simulink model "AntriebeW_V2_Heatflow_D"  (Simulink 7.6)
settings: Solver=ode45  StartTime=0.0  StopTime=SimulTime  RelTol=1e-3
values from neighbouring files (symbols this model uses):
  hsp = 200    [ParamtersAntriebeW_D.m]
  r = 0.2    [ParamtersAntriebeW_D.m]
  R = 25    [ParamtersAntriebeW_D.m]    (also in PlottingAntriebeHeatFlow.m = Scp_DrivesT.signals(3).values(:,1))
  sb = 5.67*(10^-8)    (= 5.67e-08)    [ParamtersAntriebeW_D.m]
  T_amb = 296    [ParamtersAntriebeW_D.m]
undefined symbols (not defined in the file or in its folder): A, Drive, Job, magnitude
libraries: simulink x1
settings Model: Creator=Coni  LastModifiedBy=conid

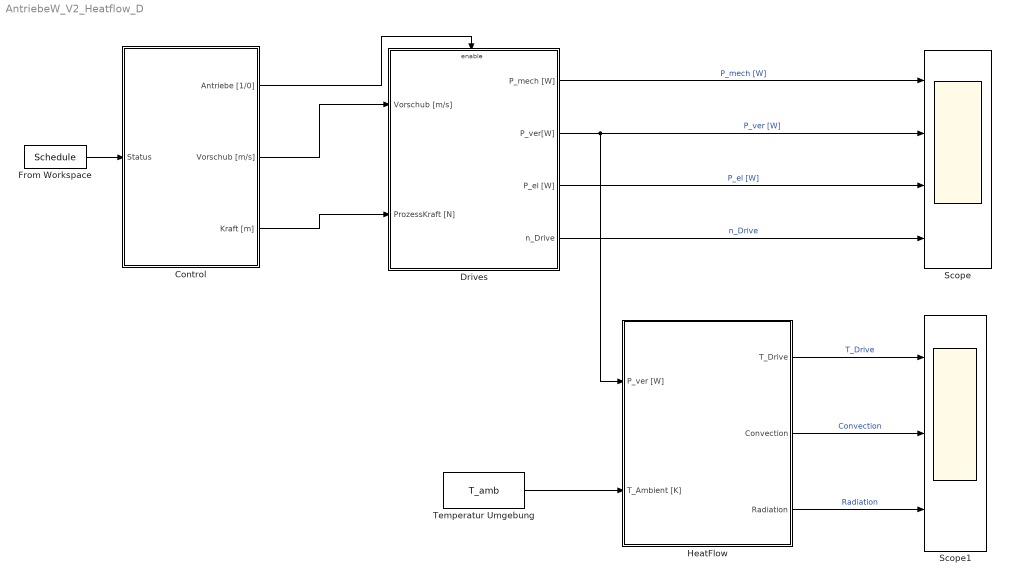
== system AntriebeW_V2_Heatflow_D ==
  Control : Subsystem  TreatAsAtomicUnit=on  mask{Antriebe=[0 1 1 1 1], Job=Job}
      mask prompts: Job "Job Struct"
      mask help:
      | Controls the components of the machine:
      |
      | Status:
      |     0. Off
      |     1. Standby
      |     2. Warmup
      |     3. Setting
      |     4. Machining
      |
      | If the status is machining, the job defined as
      |     - Job.time
      |     - Job.omega_dem
      |     - Job.M_dem
      | will be runned, and repeated.
      mask TabNameString: Status,Job
  Drives : Subsystem  TreatAsAtomicUnit=on
  From Workspace : FromWorkspace  VariableName=Schedule  SampleTime=0  Interpolate=off  OutputAfterFinalValue=Holding final value
  HeatFlow : Subsystem  TreatAsAtomicUnit=on
  Scope : Scope  NumInputPorts=4
      settings: TickLabels=on  TimeRange=2  YMin=0.014~0.036~0.022~0.3705  YMax=0.01575~0.0405~0.0245~0.4095  SaveName=Scp_Drives
  Scope1 : Scope  NumInputPorts=3
      settings: YMin=281.2~-1e-012~0  YMax=310.8~0~250  SaveName=Scp_DrivesT
  Temperatur Umgebung : Constant  Value=T_amb
  wires:
  Drives/1(P_mech [W]) -> Scope/1  "P_mech [W]"
  Drives/2(P_ver[W]) -> HeatFlow/1(P_ver [W]), Scope/2  "P_ver [W]"
  Drives/4(n_Drive) -> Scope/4  "n_Drive"
  Temperatur Umgebung/1 -> HeatFlow/2(T_Ambient [K])
  HeatFlow/1(T_Drive) -> Scope1/1  "T_Drive"
  HeatFlow/2(Convection) -> Scope1/2  "Convection"
  HeatFlow/3(Radiation) -> Scope1/3  "Radiation"
  Drives/3(P_el [W]) -> Scope/3  "P_el [W]"
  From Workspace/1 -> Control/1(Status)
  Control/2(Vorschub [m/s]) -> Drives/1(Vorschub [m/s])
  Control/3(Kraft [m]) -> Drives/2(ProzessKraft [N])
  Control/1(Antriebe [1/0]) -> Drives/Enable

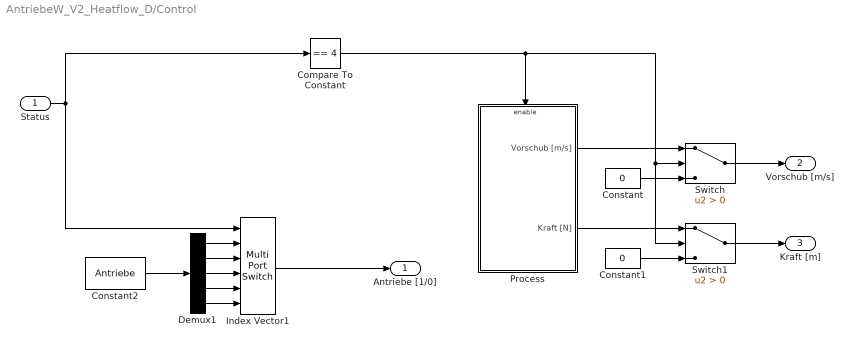
== system AntriebeW_V2_Heatflow_D/Control ==
  Status : Inport
  Compare To Constant : simulink/Logic and Bit Operations/Compare To Constant  SystemSampleTime=-1  relop===  const=4  LogicOutDataTypeMode=uint8
  Constant : Constant  Value=0
  Constant1 : Constant  Value=0
  Constant2 : Constant  Value=Antriebe
  Demux1 : Demux  Outputs=5
  Index Vector1 : MultiPortSwitch  DataPortOrder=Zero-based contiguous  Inputs=5  zeroidx=on
  Process : Subsystem  TreatAsAtomicUnit=on
  Switch : Switch  Criteria=u2 > Threshold
  Switch1 : Switch  Criteria=u2 > Threshold
  Antriebe [1/0] : Outport
  Vorschub [m/s] : Outport  Port=2
  Kraft [m] : Outport  Port=3
  wires:
  Status/1 -> Compare To Constant/1, Index Vector1/1
  Demux1/1 -> Index Vector1/2
  Demux1/2 -> Index Vector1/3
  Demux1/3 -> Index Vector1/4
  Demux1/4 -> Index Vector1/5
  Demux1/5 -> Index Vector1/6
  Index Vector1/1 -> Antriebe [1/0]/1
  Compare To Constant/1 -> Process/Enable, Switch1/2, Switch/2
  Process/1(Vorschub [m/s]) -> Switch/1
  Constant/1 -> Switch/3
  Process/2(Kraft [N]) -> Switch1/1
  Constant1/1 -> Switch1/3
  Switch/1 -> Vorschub [m/s]/1
  Switch1/1 -> Kraft [m]/1
  Constant2/1 -> Demux1/1

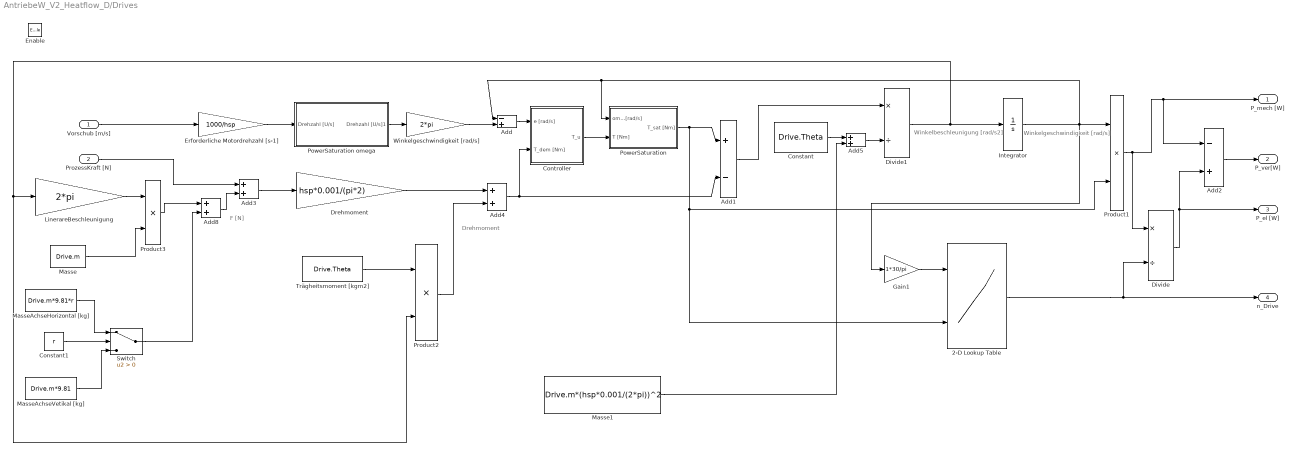
== system AntriebeW_V2_Heatflow_D/Drives ==
  note: Winkelgeschwindigkeit [rad/s]
  note: Drehmoment
  note: F [N]
  note: Winkelbeschleunigung [rad/s2]
  Vorschub [m/s] : Inport
  ProzessKraft [N] : Inport  Port=2
  Enable : EnablePort
  2-D Lookup Table : Lookup_n-D  BreakpointsForDimension1=Drive.Tabelomega  BreakpointsForDimension2=Drive.TabelM  BreakpointsForDimension1Min=[0]  BreakpointsForDimension2Min=[0]  BreakpointsForDimension1Max=[3000]  BreakpointsForDimension2Max=[9.5]  Table=Drive.Tabeleta  TableMin=[0]  TableMax=[1]  InterpMethod=Cubic spline  ExtrapMethod=None - Clip  OutMin=[0]  OutMax=[1]  RndMeth=Simplest  InputSameDT=on
  Add : Sum  Inputs=-+
  Add1 : Sum  Inputs=+-
  Add2 : Sum  Inputs=-+
  Add{3..5,8} (4 alike) : Sum
  Constant : Constant  Value=Drive.Theta
  Constant1 : Constant  Value=r
  Controller : Subsystem  TreatAsAtomicUnit=on
  Divide : Product  Inputs=*/
  Divide1 : Product  Inputs=*/
  Drehmoment : Gain  Gain=hsp*0.001/(pi*2)
  Erforderliche Motordrehzahl [s-1] : Gain  Gain=1000/hsp
  Gain1 : Gain  Gain=1*30/pi
  Integrator : Integrator
  LinerareBeschleunigung : Gain  Gain=2*pi
  Masse : Constant  Value=Drive.m
  Masse1 : Constant  Value=Drive.m*(hsp*0.001/(2*pi))^2
  MasseAchseHorizontal [kg] : Constant  Value=Drive.m*9.81*r
  MasseAchseVetikal [kg] : Constant  Value=Drive.m*9.81
  PowerSaturation : Subsystem  TreatAsAtomicUnit=on
  PowerSaturation omega : Subsystem  TreatAsAtomicUnit=on
  Product1 : Product  RndMeth=Zero
  Product2 : Product  RndMeth=Zero
  Product3 : Product  RndMeth=Zero
  Switch : Switch  Criteria=u2 > Threshold
  Trägheitsmoment [kgm2] : Constant  Value=Drive.Theta
  Winkelgeschwindigkeit [rad/s] : Gain  Gain=2*pi
  P_mech [W] : Outport
  P_ver[W] : Outport  Port=2
  P_el [W] : Outport  Port=3
  n_Drive : Outport  Port=4
  wires:
  Add/1 -> Controller/1(e [rad/s])
  Controller/1(T_u) -> PowerSaturation/2(T [Nm])
  PowerSaturation/1(T_sat [Nm]) -> Add1/1, Product1/2, 2-D Lookup Table/2
  Divide1/1 -> Integrator/1, Product2/2, LinerareBeschleunigung/1
  Integrator/1 -> Add/1, PowerSaturation/1(omega [rad/s]), Gain1/1, Product1/1
  Product1/1 -> Divide/1, P_mech [W]/1, Add2/1
  Add2/1 -> P_ver[W]/1
  Divide/1 -> Add2/2, P_el [W]/1
  Gain1/1 -> 2-D Lookup Table/1
  Add1/1 -> Divide1/1
  Add3/1 -> Drehmoment/1
  Add4/1 -> Add1/2, Controller/2(T_dem [Nm])
  Drehmoment/1 -> Add4/1
  ProzessKraft [N]/1 -> Add3/1
  Add5/1 -> Divide1/2
  Constant/1 -> Add5/1
  Trägheitsmoment [kgm2]/1 -> Product2/1
  Product2/1 -> Add4/2
  MasseAchseHorizontal [kg]/1 -> Switch/1
  MasseAchseVetikal [kg]/1 -> Switch/3
  Constant1/1 -> Switch/2
  Vorschub [m/s]/1 -> Erforderliche Motordrehzahl [s-1]/1
  Masse1/1 -> Add5/2
  Add8/1 -> Add3/2
  Switch/1 -> Add8/2
  Masse/1 -> Product3/2
  Product3/1 -> Add8/1
  LinerareBeschleunigung/1 -> Product3/1
  2-D Lookup Table/1 -> Divide/2, n_Drive/1
  Winkelgeschwindigkeit [rad/s]/1 -> Add/2
  PowerSaturation omega/1(Drehzahl [U/s]1) -> Winkelgeschwindigkeit [rad/s]/1
  Erforderliche Motordrehzahl [s-1]/1 -> PowerSaturation omega/1(Drehzahl [U/s])

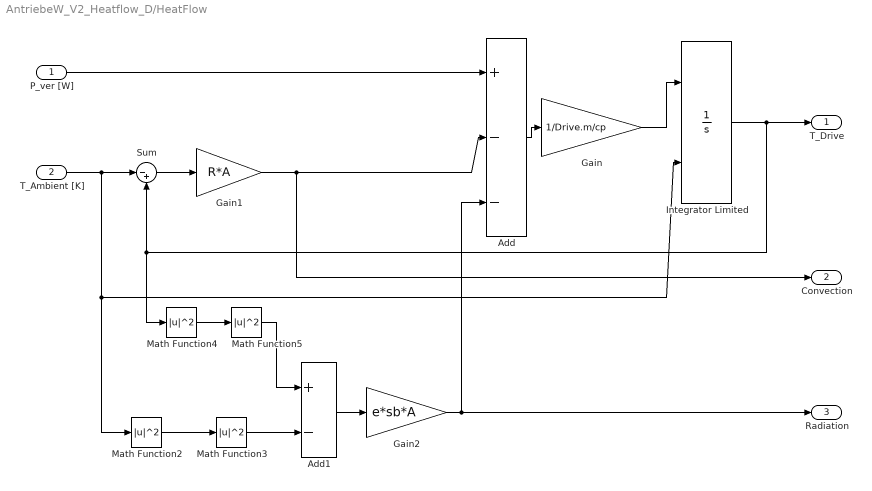
== system AntriebeW_V2_Heatflow_D/HeatFlow ==
  P_ver [W] : Inport
  T_Ambient [K] : Inport  Port=2
  Add : Sum  Inputs=+--
  Add1 : Sum  Inputs=+-
  Gain : Gain  Gain=1/Drive.m/cp
  Gain1 : Gain  Gain=R*A
  Gain2 : Gain  Gain=e*sb*A
  Integrator Limited : Integrator  InitialConditionSource=external  LimitOutput=on  ZeroCross=off
  Math Function{2..5} (4 alike) : Math  Operator=magnitude^2  SaturateOnIntegerOverflow=on
  Sum : Sum  Inputs=|-+
  T_Drive : Outport
  Convection : Outport  Port=2
  Radiation : Outport  Port=3
  wires:
  P_ver [W]/1 -> Add/1
  T_Ambient [K]/1 -> Sum/1, Integrator Limited/2, Math Function2/1
  Sum/1 -> Gain1/1
  Gain/1 -> Integrator Limited/1
  Gain1/1 -> Add/2, Convection/1
  Integrator Limited/1 -> T_Drive/1, Sum/2, Math Function4/1
  Add/1 -> Gain/1
  Gain2/1 -> Add/3, Radiation/1
  Math Function2/1 -> Math Function3/1
  Math Function4/1 -> Math Function5/1
  Math Function5/1 -> Add1/1
  Math Function3/1 -> Add1/2
  Add1/1 -> Gain2/1

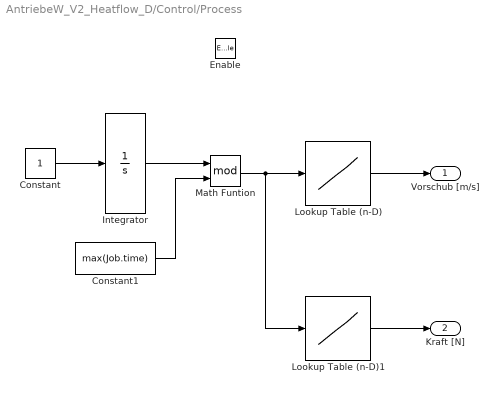
== system AntriebeW_V2_Heatflow_D/Control/Process ==
  Enable : EnablePort
  Constant : Constant
  Constant1 : Constant  Value=max(Job.time)
  Integrator : Integrator
  Lookup Table (n-D) : Lookup_n-D  NumberOfTableDimensions=1  BreakpointsForDimension1=Job.time  Table=Job.omega_dem  InterpMethod=None - Flat  ExtrapMethod=Cubic spline  InputSameDT=on
  Lookup Table (n-D)1 : Lookup_n-D  NumberOfTableDimensions=1  BreakpointsForDimension1=Job.time  Table=Job.M_dem  InterpMethod=None - Flat  InputSameDT=on
  Math Funtion : Math  Operator=mod  SaturateOnIntegerOverflow=on
  Vorschub [m/s] : Outport
  Kraft [N] : Outport  Port=2
  wires:
  Constant/1 -> Integrator/1
  Integrator/1 -> Math Funtion/1
  Math Funtion/1 -> Lookup Table (n-D)/1, Lookup Table (n-D)1/1
  Lookup Table (n-D)/1 -> Vorschub [m/s]/1
  Lookup Table (n-D)1/1 -> Kraft [N]/1
  Constant1/1 -> Math Funtion/2

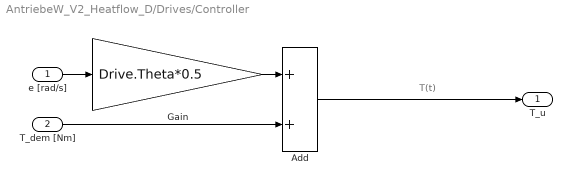
== system AntriebeW_V2_Heatflow_D/Drives/Controller ==
  note: T(t)
  e [rad/s] : Inport
  T_dem [Nm] : Inport  Port=2
  Add : Sum
  Gain : Gain  Gain=Drive.Theta*0.5
  T_u : Outport
  wires:
  Add/1 -> T_u/1
  T_dem [Nm]/1 -> Add/2
  Gain/1 -> Add/1
  e [rad/s]/1 -> Gain/1

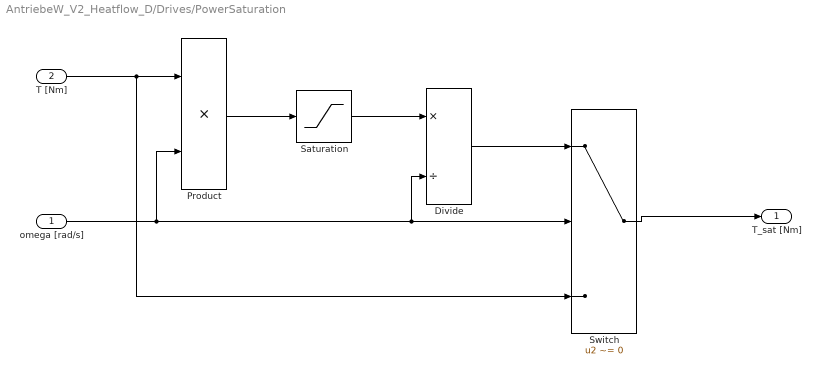
== system AntriebeW_V2_Heatflow_D/Drives/PowerSaturation ==
  omega [rad/s] : Inport
  T [Nm] : Inport  Port=2
  Divide : Product  Inputs=*/
  Product : Product  RndMeth=Zero
  Saturation : Saturate  UpperLimit=Drive.Pmax  LowerLimit=-Drive.Pmax  ZeroCross=off
  Switch : Switch  Criteria=u2 ~= 0
  T_sat [Nm] : Outport
  wires:
  Product/1 -> Saturation/1
  Saturation/1 -> Divide/1
  Divide/1 -> Switch/1
  Switch/1 -> T_sat [Nm]/1
  T [Nm]/1 -> Product/1, Switch/3
  omega [rad/s]/1 -> Switch/2, Divide/2, Product/2

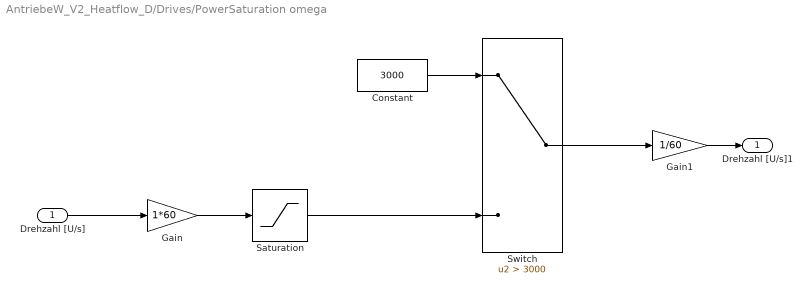
== system AntriebeW_V2_Heatflow_D/Drives/PowerSaturation omega ==
  Drehzahl [U/s] : Inport
  Constant : Constant  Value=3000
  Gain : Gain  Gain=1*60
  Gain1 : Gain  Gain=1/60
  Saturation : Saturate  UpperLimit=3000  LowerLimit=0  ZeroCross=off
  Switch : Switch  Criteria=u2 > Threshold  Threshold=3000
  Drehzahl [U/s]1 : Outport
  wires:
  Saturation/1 -> Switch/3
  Constant/1 -> Switch/1
  Drehzahl [U/s]/1 -> Gain/1
  Gain/1 -> Saturation/1
  Gain1/1 -> Drehzahl [U/s]1/1
  Switch/1 -> Gain1/1
